simulink model "SmithPredictorTheoretical"  (R2017b)
settings: Solver=VariableStepAuto  StartTime=0.0  StopTime=60.0  RelTol=1e-3
undefined symbols (not defined in the file or in its folder): s
libraries: cstblocks x6
settings Model: Creator=k37107  LastModifiedBy=k37107

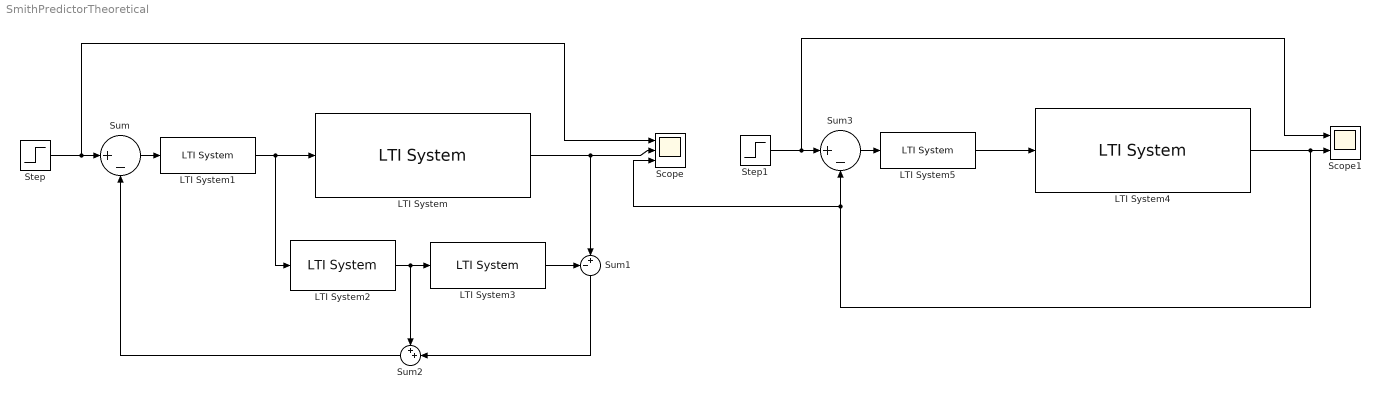
== system SmithPredictorTheoretical ==
  LTI System : cstblocks/LTI System  sys=2/(10*s+1)*exp(-5*s)  IC=[]
  LTI System1 : cstblocks/LTI System  sys=(6*(1+(1/(10*s))))  IC=[]
  LTI System2 : cstblocks/LTI System  sys=2/(10*s+1)  IC=[]
  LTI System3 : cstblocks/LTI System  sys=exp(-5*s)  IC=[]
  LTI System4 : cstblocks/LTI System  sys=2/(10*s+1)*exp(-5*s)  IC=[]
  LTI System5 : cstblocks/LTI System  sys=(0.56*(1+(1/(10*s))))  IC=[]
  Scope : Scope  NumInputPorts=3
  Scope1 : Scope  NumInputPorts=2
  Step : Step  After=5  SampleTime=0
  Step1 : Step  After=5  SampleTime=0
  Sum : Sum  Inputs=|+-
  Sum1 : Sum  Inputs=-+|
  Sum2 : Sum  Inputs=++|
  Sum3 : Sum  Inputs=|+-
  wires:
  Step/1 -> Scope/1, Sum/1
  Sum/1 -> LTI System1/1
  LTI System/1 -> Sum1/2, Scope/2
  LTI System1/1 -> LTI System2/1, LTI System/1
  LTI System3/1 -> Sum1/1
  LTI System2/1 -> Sum2/1, LTI System3/1
  Sum1/1 -> Sum2/2
  Sum2/1 -> Sum/2
  Step1/1 -> Scope1/1, Sum3/1
  Sum3/1 -> LTI System5/1
  LTI System5/1 -> LTI System4/1
  LTI System4/1 -> Scope/3, Sum3/2, Scope1/2
